simulink model "psk"  (R2018b)
settings: Solver=VariableStepAuto  StartTime=0.0  StopTime=10.0  RelTol=1e-3
libraries: dsparch4 x2, commchan3 x1, commrandsrc3 x1
settings Model: Creator=lance  LastModifiedBy=lance

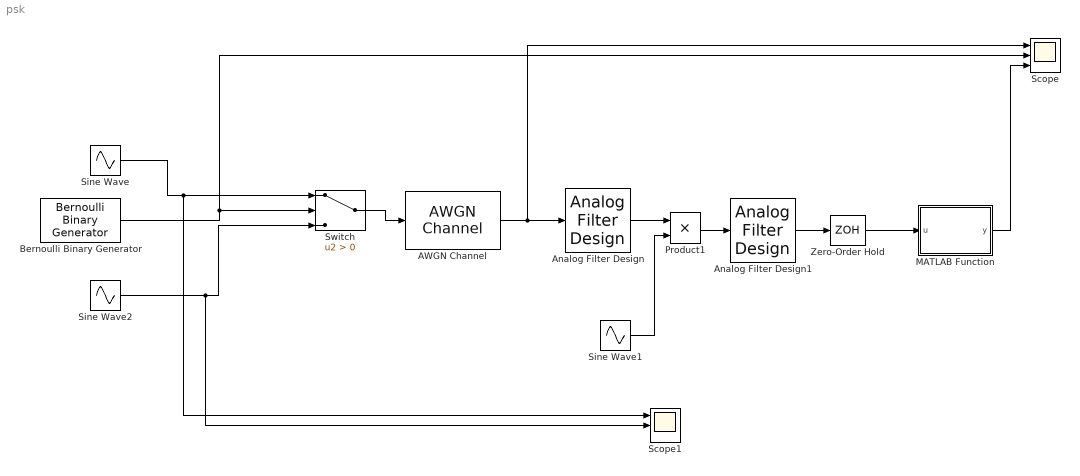
== system psk ==
  AWGN Channel : commchan3/AWGN Channel  InputProcessing=Columns as channels (frame based)  seed=61  noiseMode="Signal to noise ratio  (SNR)"  EbNodB=10  EsNodB=10  SNRdB=10  bitsPerSym=1  Ps=1  Tsym=1  variance=1
  Analog Filter Design : dsparch4/Analog Filter Design  method=Butterworth  filttype=Bandpass  N=8  Wlo=97*2*pi  Whi=103*2*pi  Rp=2  Rs=40
  Analog Filter Design1 : dsparch4/Analog Filter Design  method=Butterworth  filttype=Lowpass  N=8  Wlo=10*2*pi  Whi=103*2*pi  Rp=2  Rs=40
  Bernoulli Binary Generator : commrandsrc3/Bernoulli Binary Generator  ProbabilityOfZero=0.5  SeedSource=Parameter  Seed=61  SampleTime=0.1  SamplesPerFrame=1  OutputDataType=double  SimulateUsing=Interpreted execution
  MATLAB Function : MATLAB Function  TreatAsAtomicUnit=on
  Product1 : Product
  Scope : Scope  NumInputPorts=3
  Scope1 : Scope  NumInputPorts=3
  Sine Wave : Sin  Frequency=100*2*pi  SampleTime=0.0001
  Sine Wave1 : Sin  Frequency=100*2*pi  SampleTime=0.0001
  Sine Wave2 : Sin  Frequency=100*2*pi  Phase=pi  SampleTime=0.0001
  Switch : Switch  Criteria=u2 > Threshold
  Zero-Order Hold : ZeroOrderHold  SampleTime=0.01
  wires:
  Sine Wave1/1 -> Product1/2
  Zero-Order Hold/1 -> MATLAB Function/1(u)
  Bernoulli Binary Generator/1 -> Switch/2, Scope/2
  Sine Wave/1 -> Scope1/1, Switch/1
  Analog Filter Design/1 -> Product1/1
  Product1/1 -> Analog Filter Design1/1
  Analog Filter Design1/1 -> Zero-Order Hold/1
  Sine Wave2/1 -> Scope1/2, Switch/3
  Switch/1 -> AWGN Channel/1
  AWGN Channel/1 -> Scope/1, Analog Filter Design/1
  MATLAB Function/1(y) -> Scope/3

== matlab function psk/MATLAB Function ==
  data: u input; y output
function y = fcn(u)
if(u>0)
    y=1;
else
    y=0;
end
